simulink model "sistem_ver"  (R2020b)
settings: Solver=ode45  StartTime=0.0  StopTime=10  MaxStep=0.01  RelTol=1e-3
undefined symbols (not defined in the file or in its folder): K_d, K_p, params, r_des
settings Model: Creator=Danil  LastModifiedBy=Danil

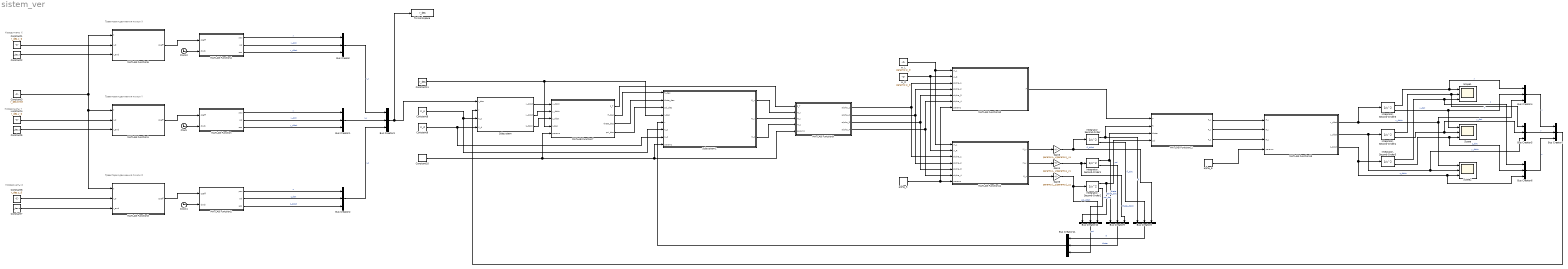
== system sistem_ver ==
  note: Траектория движения по оси Z
  note: Траектория движения по оси Y
  note: Координаты Y
  note: Траектория движения по оси X
  note: Координаты Z
  note: Координаты X
  Bus Creator{,1..11} (12 alike) : BusCreator  Inputs=3
  Clock : Clock
  Clock1 : Clock
  Clock2 : Clock
  Constant1 : Constant  Value=r_des.x_0
  Constant10 : Constant  Value=params  OutDataTypeStr=Bus: params_bus
  Constant11 : Constant  Value=r_des  OutDataTypeStr=Bus: r_des_bus
  Constant2 : Constant  Value=r_des.x
  Constant3 : Constant  Value=r_des.time
  Constant4 : Constant  Value=r_des.y_0
  Constant5 : Constant  Value=r_des.y
  Constant6 : Constant  Value=r_des.z_0
  Constant7 : Constant  Value=r_des.z
  Constant8 : Constant  Value=K_p  OutDataTypeStr=Bus: K_p_bus
  Constant9 : Constant  Value=K_d  OutDataTypeStr=Bus: K_d_bus
  Gain3 : Gain  Gain=params.L_x/params.J_xx
  Gain4 : Gain  Gain=params.L_y/params.J_yy
  Gain5 : Gain  Gain=params.L_z/params.J_zz
  Integrator, Second-Order{,1..5} (6 alike) : SecondOrderIntegrator
  MATLAB Function : MATLAB Function  TreatAsAtomicUnit=on
  MATLAB Function1 : MATLAB Function  TreatAsAtomicUnit=on
  MATLAB Function10 : MATLAB Function  TreatAsAtomicUnit=on
  MATLAB Function11 : MATLAB Function  TreatAsAtomicUnit=on
  MATLAB Function12 : MATLAB Function  TreatAsAtomicUnit=on
  MATLAB Function13 : MATLAB Function  TreatAsAtomicUnit=on
  MATLAB Function2 : MATLAB Function  TreatAsAtomicUnit=on
  MATLAB Function3 : MATLAB Function  TreatAsAtomicUnit=on
  MATLAB Function4 : MATLAB Function  TreatAsAtomicUnit=on
  MATLAB Function5 : MATLAB Function  TreatAsAtomicUnit=on
  MATLAB Function7 : MATLAB Function  TreatAsAtomicUnit=on
  MATLAB Function9 : MATLAB Function  TreatAsAtomicUnit=on
  Scope : Scope  NumInputPorts=3
  Scope1 : Scope  NumInputPorts=3
  Scope2 : Scope  NumInputPorts=3
  Subsystem : Subsystem
  Subsystem1 : Subsystem
  To Workspace : ToWorkspace  VariableName=r_des  SaveFormat=Timeseries  SampleTime=-1
  alpha_5 : Constant  Value=params  OutDataTypeStr=Bus: params_bus
  alpha_6 : Constant  Value=params  OutDataTypeStr=Bus: params_bus
  w_L : Constant  Value=params.w_0
  w_R : Constant  Value=params.w_0
  wires:
  MATLAB Function/3(acc) -> Bus Creator1/3  "y_ddot"
  Bus Creator/1 -> Bus Creator3/1  "r_x"
  MATLAB Function2/3(acc) -> Bus Creator2/3  "z_ddot"
  Bus Creator1/1 -> Bus Creator3/2  "r_y"
  Bus Creator2/1 -> Bus Creator3/3  "r_z"
  MATLAB Function3/1(coeff) -> MATLAB Function2/1(coeff)
  Clock/1 -> MATLAB Function/2(clock)
  Constant4/1 -> MATLAB Function1/2(r_0)
  Clock1/1 -> MATLAB Function2/2(clock)
  MATLAB Function1/1(coeff) -> MATLAB Function/1(coeff)
  Constant3/1 -> MATLAB Function3/1(t), MATLAB Function1/1(t), MATLAB Function5/1(t)
  Constant5/1 -> MATLAB Function1/3(r_end)
  Constant2/1 -> MATLAB Function5/3(r_end)
  Constant1/1 -> MATLAB Function5/2(r_0)
  MATLAB Function2/1(pos) -> Bus Creator2/1  "z"
  MATLAB Function/1(pos) -> Bus Creator1/1  "y"
  Constant7/1 -> MATLAB Function3/3(r_end)
  Constant6/1 -> MATLAB Function3/2(r_0)
  MATLAB Function/2(vel) -> Bus Creator1/2  "y_dot"
  MATLAB Function5/1(coeff) -> MATLAB Function4/1(coeff)
  Clock2/1 -> MATLAB Function4/2(clock)
  MATLAB Function4/2(vel) -> Bus Creator/2  "x_dot"
  MATLAB Function4/3(acc) -> Bus Creator/3  "x_ddot"
  MATLAB Function4/1(pos) -> Bus Creator/1  "x"
  MATLAB Function2/2(vel) -> Bus Creator2/2  "z_dot"
  MATLAB Function7/1(F_T) -> MATLAB Function9/1(F_T)
  Constant10/1 -> MATLAB Function7/5(params), Subsystem1/8(params), MATLAB Function9/5(params)
  "Integrator, Second-Order"/1 -> Bus Creator8/1, MATLAB Function12/2(fi)  "fi"
  MATLAB Function11/3(M_z) -> Gain5/1
  "Integrator, Second-Order2"/1 -> Bus Creator10/1, MATLAB Function12/4(psi)  "psi"
  "Integrator, Second-Order5"/2 -> Bus Creator6/2, Scope/3  "z_dot"
  Gain5/1 -> "Integrator, Second-Order2"/1, Bus Creator10/3  "psi_ddot"
  "Integrator, Second-Order4"/2 -> Bus Creator5/2, Scope/2  "y_dot"
  MATLAB Function11/2(M_y) -> Gain4/1
  w_R/1 -> MATLAB Function11/2(w_R), MATLAB Function10/2(w_R)
  "Integrator, Second-Order5"/1 -> Bus Creator6/1, Scope1/3  "z"
  MATLAB Function12/2(F_y) -> MATLAB Function13/2(F_y)
  MATLAB Function12/1(F_x) -> MATLAB Function13/1(F_x)
  "Integrator, Second-Order3"/2 -> Bus Creator4/2, Scope/1  "x_dot"
  MATLAB Function13/1(x_ddot) -> "Integrator, Second-Order3"/1, Bus Creator4/3, Scope2/1  "x_ddot"
  "Integrator, Second-Order3"/1 -> Bus Creator4/1, Scope1/1  "x"
  MATLAB Function13/3(z_ddot) -> Bus Creator6/3, Scope2/3, "Integrator, Second-Order5"/1  "z_ddot"
  MATLAB Function13/2(y_ddot) -> Bus Creator5/3, Scope2/2, "Integrator, Second-Order4"/1  "y_ddot"
  "Integrator, Second-Order1"/1 -> Bus Creator9/1, MATLAB Function12/3(theta)  "theta"
  MATLAB Function11/1(M_x) -> Gain3/1
  alpha_5/1 -> MATLAB Function10/7(params), MATLAB Function11/7(params)
  "Integrator, Second-Order4"/1 -> Bus Creator5/1, Scope1/2  "y"
  MATLAB Function9/3(alpha_3) -> MATLAB Function11/5(alpha_3), MATLAB Function10/5(alpha_3)
  alpha_6/1 -> MATLAB Function13/4(params)
  w_L/1 -> MATLAB Function10/1(w_L), MATLAB Function11/1(w_L)
  Gain3/1 -> Bus Creator8/3, "Integrator, Second-Order"/1  "fi_ddot"
  Gain4/1 -> Bus Creator9/3, "Integrator, Second-Order1"/1  "theta_ddot"
  MATLAB Function9/2(alpha_2) -> MATLAB Function11/4(alpha_2), MATLAB Function10/4(alpha_2)
  MATLAB Function9/1(alpha_1) -> MATLAB Function10/3(alpha_1), MATLAB Function11/3(alpha_1)
  MATLAB Function10/1(F) -> MATLAB Function12/1(F)
  MATLAB Function12/3(F_z) -> MATLAB Function13/3(F_z)
  MATLAB Function9/4(alpha_4) -> MATLAB Function11/6(alpha_4), MATLAB Function10/6(alpha_4)
  Constant8/1 -> Subsystem1/6(K_p), Subsystem/3(K_p)
  Constant9/1 -> Subsystem1/7(K_d), Subsystem/4(K_d)
  Bus Creator3/1 -> To Workspace/1, Subsystem/1(r_des)
  Constant11/1 -> MATLAB Function7/4(r_des), Subsystem1/4(r_des)
  "Integrator, Second-Order"/2 -> Bus Creator8/2  "fi_dot"
  "Integrator, Second-Order1"/2 -> Bus Creator9/2  "tehta_dot"
  "Integrator, Second-Order2"/2 -> Bus Creator10/2  "psi_dot"
  Bus Creator9/1 -> Bus Creator11/2  "theta"
  Bus Creator8/1 -> Bus Creator11/1  "fi"
  Bus Creator10/1 -> Bus Creator11/3  "psi"
  Bus Creator4/1 -> Bus Creator7/1  "x"
  Bus Creator5/1 -> Bus Creator7/2  "y"
  Bus Creator6/1 -> Bus Creator7/3  "z"
  Bus Creator7/1 -> Subsystem/2(r)
  Subsystem/1(x_ddot) -> MATLAB Function7/1(x_ddot)
  Subsystem/2(y_ddot) -> MATLAB Function7/2(y_ddot)
  Subsystem/3(z_ddot) -> MATLAB Function7/3(z_ddot)
  MATLAB Function7/2(fi_des) -> Subsystem1/1(fi_des)
  MATLAB Function7/3(theta_des) -> Subsystem1/2(theta_des)
  MATLAB Function7/4(psi_des) -> Subsystem1/3(psi_des)
  Bus Creator11/1 -> Subsystem1/5(r)
  Subsystem1/1(M_x) -> MATLAB Function9/2(M_x)
  Subsystem1/2(M_y) -> MATLAB Function9/3(M_y)
  Subsystem1/3(M_z) -> MATLAB Function9/4(M_z)

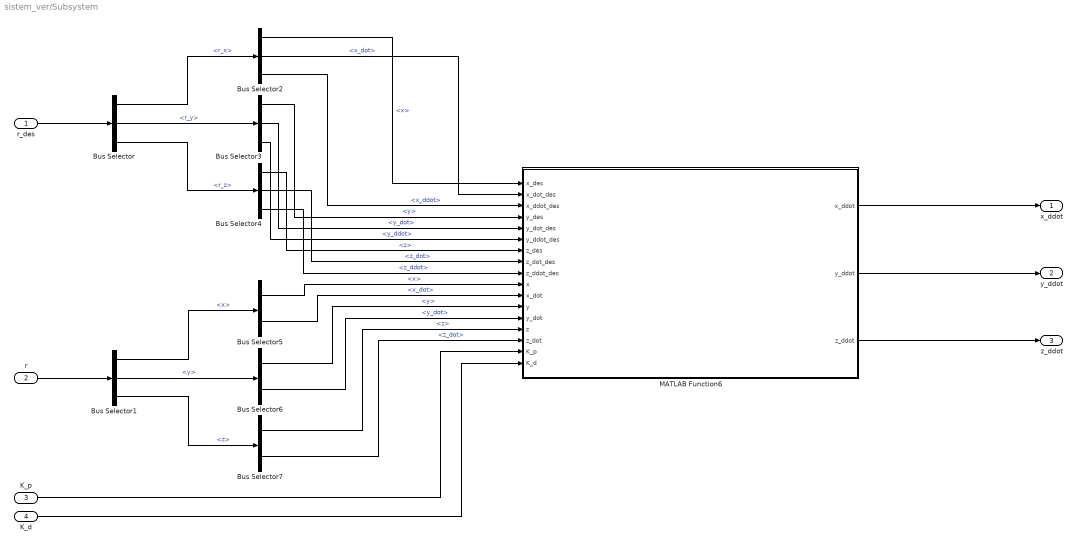
== system sistem_ver/Subsystem ==
  r_des : Inport
  r : Inport  Port=2
  K_p : Inport  Port=3
  K_d : Inport  Port=4
  Bus Selector : BusSelector  OutputSignals=r_x,r_y,r_z
  Bus Selector1 : BusSelector  OutputSignals=x,y,z
  Bus Selector2 : BusSelector  OutputSignals=x,x_dot,x_ddot
  Bus Selector3 : BusSelector  OutputSignals=y,y_dot,y_ddot
  Bus Selector4 : BusSelector  OutputSignals=z,z_dot,z_ddot
  Bus Selector5 : BusSelector  OutputSignals=x,x_dot
  Bus Selector6 : BusSelector  OutputSignals=y,y_dot
  Bus Selector7 : BusSelector  OutputSignals=z,z_dot
  MATLAB Function6 : MATLAB Function  TreatAsAtomicUnit=on
  x_ddot : Outport
  y_ddot : Outport  Port=2
  z_ddot : Outport  Port=3
  wires:
  MATLAB Function6/1(x_ddot) -> x_ddot/1
  MATLAB Function6/3(z_ddot) -> z_ddot/1
  K_p/1 -> MATLAB Function6/16(K_p)
  MATLAB Function6/2(y_ddot) -> y_ddot/1
  K_d/1 -> MATLAB Function6/17(K_d)
  r_des/1 -> Bus Selector/1
  r/1 -> Bus Selector1/1
  Bus Selector/1 -> Bus Selector2/1  "<r_x>"
  Bus Selector/2 -> Bus Selector3/1  "<r_y>"
  Bus Selector/3 -> Bus Selector4/1  "<r_z>"
  Bus Selector1/1 -> Bus Selector5/1  "<x>"
  Bus Selector1/2 -> Bus Selector6/1  "<y>"
  Bus Selector1/3 -> Bus Selector7/1  "<z>"
  Bus Selector2/1 -> MATLAB Function6/1(x_des)  "<x>"
  Bus Selector2/2 -> MATLAB Function6/2(x_dot_des)  "<x_dot>"
  Bus Selector2/3 -> MATLAB Function6/3(x_ddot_des)  "<x_ddot>"
  Bus Selector3/1 -> MATLAB Function6/4(y_des)  "<y>"
  Bus Selector3/2 -> MATLAB Function6/5(y_dot_des)  "<y_dot>"
  Bus Selector3/3 -> MATLAB Function6/6(y_ddot_des)  "<y_ddot>"
  Bus Selector4/1 -> MATLAB Function6/7(z_des)  "<z>"
  Bus Selector4/2 -> MATLAB Function6/8(z_dot_des)  "<z_dot>"
  Bus Selector4/3 -> MATLAB Function6/9(z_ddot_des)  "<z_ddot>"
  Bus Selector5/1 -> MATLAB Function6/10(x)  "<x>"
  Bus Selector5/2 -> MATLAB Function6/11(x_dot)  "<x_dot>"
  Bus Selector6/1 -> MATLAB Function6/12(y)  "<y>"
  Bus Selector6/2 -> MATLAB Function6/13(y_dot)  "<y_dot>"
  Bus Selector7/1 -> MATLAB Function6/14(z)  "<z>"
  Bus Selector7/2 -> MATLAB Function6/15(z_dot)  "<z_dot>"

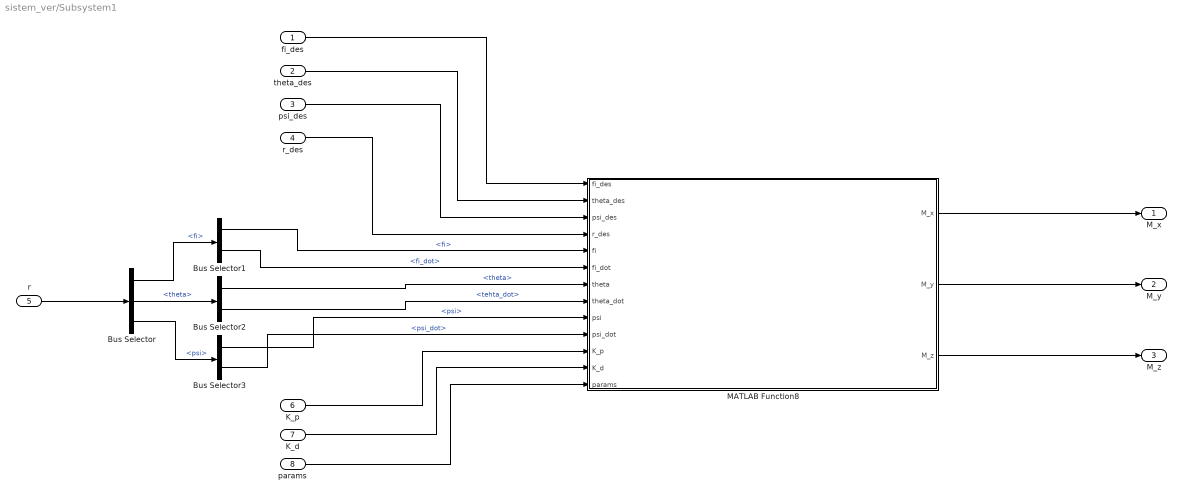
== system sistem_ver/Subsystem1 ==
  fi_des : Inport
  theta_des : Inport  Port=2
  psi_des : Inport  Port=3
  r_des : Inport  Port=4
  r : Inport  Port=5
  K_p : Inport  Port=6
  K_d : Inport  Port=7
  params : Inport  Port=8
  Bus Selector : BusSelector  OutputSignals=fi,theta,psi
  Bus Selector1 : BusSelector  OutputSignals=fi,fi_dot
  Bus Selector2 : BusSelector  OutputSignals=theta,tehta_dot
  Bus Selector3 : BusSelector  OutputSignals=psi,psi_dot
  MATLAB Function8 : MATLAB Function  TreatAsAtomicUnit=on
  M_x : Outport
  M_y : Outport  Port=2
  M_z : Outport  Port=3
  wires:
  MATLAB Function8/1(M_x) -> M_x/1
  params/1 -> MATLAB Function8/13(params)
  r_des/1 -> MATLAB Function8/4(r_des)
  psi_des/1 -> MATLAB Function8/3(psi_des)
  fi_des/1 -> MATLAB Function8/1(fi_des)
  theta_des/1 -> MATLAB Function8/2(theta_des)
  MATLAB Function8/2(M_y) -> M_y/1
  MATLAB Function8/3(M_z) -> M_z/1
  K_d/1 -> MATLAB Function8/12(K_d)
  K_p/1 -> MATLAB Function8/11(K_p)
  r/1 -> Bus Selector/1
  Bus Selector/1 -> Bus Selector1/1  "<fi>"
  Bus Selector/2 -> Bus Selector2/1  "<theta>"
  Bus Selector/3 -> Bus Selector3/1  "<psi>"
  Bus Selector1/1 -> MATLAB Function8/5(fi)  "<fi>"
  Bus Selector1/2 -> MATLAB Function8/6(fi_dot)  "<fi_dot>"
  Bus Selector2/1 -> MATLAB Function8/7(theta)  "<theta>"
  Bus Selector2/2 -> MATLAB Function8/8(theta_dot)  "<tehta_dot>"
  Bus Selector3/1 -> MATLAB Function8/9(psi)  "<psi>"
  Bus Selector3/2 -> MATLAB Function8/10(psi_dot)  "<psi_dot>"

== matlab function sistem_ver/MATLAB Function7 ==
  data: F_T output; fi_des output; x_ddot input; y_ddot input; z_ddot input; r_des input; params input; theta_des output; psi_des output
function [F_T, fi_des, theta_des, psi_des] = fcn(x_ddot, y_ddot, z_ddot, r_des, params)

F_T = params.m * (z_ddot + params.g);

fi_des = (1 / params.g) * (x_ddot * sin(r_des.psi) - y_ddot * cos(r_des.psi));
theta_des = (1 / params.g) * (x_ddot * cos(r_des.psi) + y_ddot * sin(r_des.psi));
psi_des = r_des.psi;

== matlab function sistem_ver/Subsystem1/MATLAB Function8 ==
  data: fi_des input; theta_des input; psi_des input; r_des input; fi input; fi_dot input; theta input; theta_dot input; psi input; psi_dot input; M_x output; K_p input; K_d input; params input; M_y output; M_z output
function [M_x, M_y, M_z] = fcn(fi_des, theta_des, psi_des, r_des, fi, fi_dot, theta, theta_dot, psi, psi_dot, K_p, K_d, params)

M_x = (params.J_xx / params.L_x) * (r_des.fi_ddot + abs(K_d.fi) * (r_des.fi_dot - fi_dot) + abs(K_p.fi) * (fi_des - fi));
M_y = (params.J_yy / params.L_y) * (r_des.theta_ddot + abs(K_d.theta) * (r_des.theta_dot - theta_dot) + abs(K_p.theta) * (theta_des - theta));
M_z = (params.J_zz / params.L_z) * (r_des.psi_ddot + abs(K_d.psi) * (r_des.psi_dot - psi_dot) + abs(K_p.psi) * (psi_des - psi));

== matlab function sistem_ver/MATLAB Function9 ==
  data: F_T input; alpha_1 output; M_x input; M_y input; M_z input; params input; alpha_2 output; alpha_3 output; alpha_4 output
function [alpha_1, alpha_2, alpha_3, alpha_4] = fcn(F_T, M_x, M_y, M_z, params)

alpha_1 = (1 / (4 * params.k_Y)) * (F_T + M_x + M_y + M_z) - 7;
alpha_2 = (1 / (4 * params.k_Y)) * (F_T + M_x - M_y - M_z);
alpha_3 = (1 / (4 * params.k_Y)) * (F_T - M_x + M_y - M_z) - 7;
alpha_4 = (1 / (4 * params.k_Y)) * (F_T - M_x - M_y + M_z);

== matlab function sistem_ver/MATLAB Function10 ==
  data: w_L input; F output; w_R input; alpha_1 input; alpha_2 input; alpha_3 input; alpha_4 input; params input
function F = fcn(w_L, w_R, alpha_1, alpha_2, alpha_3, alpha_4, params)
alpha_L = alpha_1 + alpha_2;
alpha_R = alpha_3 + alpha_4;

C_Y_L = 0.1545 * (alpha_L + 7);
C_Y_R = 0.1545 * (alpha_R + 7);

F = (3/2) * params.rho * params.S_l * (C_Y_L * w_L^2 + C_Y_R * w_R^2);

== matlab function sistem_ver/MATLAB Function11 ==
  data: w_L input; M_x output; w_R input; alpha_1 input; alpha_2 input; alpha_3 input; alpha_4 input; params input; M_y output; M_z output
function [M_x, M_y, M_z] = fcn(w_L, w_R, alpha_1, alpha_2, alpha_3, alpha_4, params)

%alpha_1 = alpha_1 * pi / 180;
%alpha_2 = alpha_2 * pi / 180;
%alpha_3 = alpha_3 * pi / 180;
%alpha_4 = alpha_4 * pi / 180;

%M_x = params.k_F * (w_L^2 * (alpha_1 + alpha_2) - w_R^2 * (alpha_3 + alpha_4));
%M_y = params.k_F * (w_L^2 * (alpha_1 - alpha_2) + w_R^2 * (alpha_3 - alpha_4));
%M_z = params.k_F * (w_L^2 * (alpha_1 - alpha_2) - w_R^2 * (alpha_3 - alpha_4));

M_x = (3/2) * params.rho * params.S_l * (0.1545 * ((alpha_1 + alpha_2) + 7) * w_L^2 - 0.1545 * ((alpha_3 + alpha_4) + 7) * w_R^2);
M_y = (3/2) * params.rho * params.S_l * (0.1545 * ((alpha_1 - alpha_2) + 7) * w_L^2 + 0.1545 * ((alpha_3 - alpha_4) + 7) * w_R^2);
M_z = (3/2) * params.rho * params.S_l * (0.1545 * ((alpha_1 - alpha_2) + 7) * w_L^2 - 0.1545 * ((alpha_3 - alpha_4) + 7) * w_R^2);

== matlab function sistem_ver/MATLAB Function12 ==
  data: F input; F_x output; fi input; theta input; psi input; F_y output; F_z output
function [F_x, F_y, F_z] = fcn(F, fi, theta, psi)

F_x = F * (cos(psi) * theta + fi * sin(psi));
F_y = F * (sin(psi) * theta - cos(psi) * fi);
F_z = F;

== matlab function sistem_ver/MATLAB Function13 ==
  data: F_x input; x_ddot output; F_y input; F_z input; params input; y_ddot output; z_ddot output
function [x_ddot, y_ddot, z_ddot] = fcn(F_x, F_y, F_z, params)

x_ddot = (1 / params.m) * F_x;
y_ddot = (1 / params.m) * F_y;
z_ddot = (1 / params.m) * (F_z - params.m * params.g);

== matlab function sistem_ver/MATLAB Function1 ==
  data: t input; coeff output; r_0 input; r_end input
function coeff  = calculation_coefficients(t, r_0, r_end)

x_0 = r_0;
x_dot_0 = 0;
x_ddot_0 = 0;

x_des = r_end;
x_dot_des = 0;
x_ddot_des = 0;

waypoints = [x_0    x_dot_0     x_ddot_0;
             x_des  x_dot_des   x_ddot_des]';
t = [0 t];

time_size = size(t);
n = 0;
%T = linspace(0, time_size(2) - 1, point(2));


border_conditions_sigm = reshape(waypoints(:, n + 1 : n + 2),1,[]);
%disp(border_conditions_sigm)

coeff = zeros(6, 1);

parameters = [1 * (t(n + 1) ^ 5), 1 * (t(n + 1) ^ 4), 1 * (t(n + 1) ^ 3), 1 * (t(n + 1) ^ 2), 1 * (t(n + 1) ^ 1), 1 * (t(n + 1) ^ 0);
              5 * (t(n + 1) ^ 4), 4 * (t(n + 1) ^ 3), 3 * (t(n + 1) ^ 2), 2 * (t(n + 1) ^ 1), 1 * (t(n + 1) ^ 0), 0 * (t(n + 1) ^ 0);
              20 * (t(n + 1) ^ 3), 12 * (t(n + 1) ^ 2), 6 * (t(n + 1) ^ 1), 2 * (t(n + 1) ^ 0), 0 * (t(n + 1) ^ 0), 0 * (t(n + 1) ^ 0);
              1 * (t(n + 2) ^ 5), 1 * (t(n + 2) ^ 4), 1 * (t(n + 2) ^ 3), 1 * (t(n + 2) ^ 2), 1 * (t(n + 2) ^ 1), 1 * (t(n + 2) ^ 0);
              5 * (t(n + 2) ^ 4), 4 * (t(n + 2) ^ 3), 3 * (t(n + 2) ^ 2), 2 * (t(n + 2) ^ 1), 1 * (t(n + 2) ^ 0), 0 * (t(n + 2) ^ 0);
              20 * (t(n + 2) ^ 3), 12 * (t(n + 2) ^ 2), 6 * (t(n + 2) ^ 1), 2 * (t(n + 2) ^ 0), 0 * (t(n + 2) ^ 0), 0 * (t(n + 2) ^ 0)];

coeff = inv(parameters) * border_conditions_sigm';

== matlab function sistem_ver/MATLAB Function ==
  data: coeff input; pos output; clock input; vel output; acc output
function [pos, vel, acc] = trajectories_calculation(coeff, clock)

T_p = [clock^5      clock^4     clock^3     clock^2     clock   1]';
T_v = [5*clock^4    4*clock^3   3*clock^2   2*clock     1       0]';
T_a = [20*clock^3   12*clock^2  6*clock     2           0       0]';

pos = sum(coeff.*T_p);
vel = sum(coeff.*T_v);
acc = sum(coeff.*T_a);

== matlab function sistem_ver/MATLAB Function2 ==
  data: coeff input; pos output; clock input; vel output; acc output
function [pos, vel, acc] = trajectories_calculation(coeff, clock)

T_p = [clock^5      clock^4     clock^3     clock^2     clock   1]';
T_v = [5*clock^4    4*clock^3   3*clock^2   2*clock     1       0]';
T_a = [20*clock^3   12*clock^2  6*clock     2           0       0]';

pos = sum(coeff.*T_p);
vel = sum(coeff.*T_v);
acc = sum(coeff.*T_a);

== matlab function sistem_ver/MATLAB Function3 ==
  data: t input; coeff output; r_0 input; r_end input
function coeff  = calculation_coefficients(t, r_0, r_end)

x_0 = r_0;
x_dot_0 = 0;
x_ddot_0 = 0;

x_des = r_end;
x_dot_des = 0;
x_ddot_des = 0;

waypoints = [x_0    x_dot_0     x_ddot_0;
             x_des  x_dot_des   x_ddot_des]';
t = [0 t];

time_size = size(t);
n = 0;
%T = linspace(0, time_size(2) - 1, point(2));


border_conditions_sigm = reshape(waypoints(:, n + 1 : n + 2),1,[]);
%disp(border_conditions_sigm)

coeff = zeros(6, 1);

parameters = [1 * (t(n + 1) ^ 5), 1 * (t(n + 1) ^ 4), 1 * (t(n + 1) ^ 3), 1 * (t(n + 1) ^ 2), 1 * (t(n + 1) ^ 1), 1 * (t(n + 1) ^ 0);
              5 * (t(n + 1) ^ 4), 4 * (t(n + 1) ^ 3), 3 * (t(n + 1) ^ 2), 2 * (t(n + 1) ^ 1), 1 * (t(n + 1) ^ 0), 0 * (t(n + 1) ^ 0);
              20 * (t(n + 1) ^ 3), 12 * (t(n + 1) ^ 2), 6 * (t(n + 1) ^ 1), 2 * (t(n + 1) ^ 0), 0 * (t(n + 1) ^ 0), 0 * (t(n + 1) ^ 0);
              1 * (t(n + 2) ^ 5), 1 * (t(n + 2) ^ 4), 1 * (t(n + 2) ^ 3), 1 * (t(n + 2) ^ 2), 1 * (t(n + 2) ^ 1), 1 * (t(n + 2) ^ 0);
              5 * (t(n + 2) ^ 4), 4 * (t(n + 2) ^ 3), 3 * (t(n + 2) ^ 2), 2 * (t(n + 2) ^ 1), 1 * (t(n + 2) ^ 0), 0 * (t(n + 2) ^ 0);
              20 * (t(n + 2) ^ 3), 12 * (t(n + 2) ^ 2), 6 * (t(n + 2) ^ 1), 2 * (t(n + 2) ^ 0), 0 * (t(n + 2) ^ 0), 0 * (t(n + 2) ^ 0)];

coeff = inv(parameters) * border_conditions_sigm';

== matlab function sistem_ver/MATLAB Function4 ==
  data: coeff input; pos output; clock input; vel output; acc output
function [pos, vel, acc] = trajectories_calculation(coeff, clock)

T_p = [clock^5      clock^4     clock^3     clock^2     clock   1]';
T_v = [5*clock^4    4*clock^3   3*clock^2   2*clock     1       0]';
T_a = [20*clock^3   12*clock^2  6*clock     2           0       0]';

pos = sum(coeff.*T_p);
vel = sum(coeff.*T_v);
acc = sum(coeff.*T_a);

== matlab function sistem_ver/MATLAB Function5 ==
  data: t input; coeff output; r_0 input; r_end input
function coeff  = calculation_coefficients(t, r_0, r_end)

x_0 = r_0;
x_dot_0 = 0;
x_ddot_0 = 0;

x_des = r_end;
x_dot_des = 0;
x_ddot_des = 0;

waypoints = [x_0    x_dot_0     x_ddot_0;
             x_des  x_dot_des   x_ddot_des]';
t = [0 t];

time_size = size(t);
n = 0;
%T = linspace(0, time_size(2) - 1, point(2));


border_conditions_sigm = reshape(waypoints(:, n + 1 : n + 2),1,[]);
%disp(border_conditions_sigm)

coeff = zeros(6, 1);

parameters = [1 * (t(n + 1) ^ 5), 1 * (t(n + 1) ^ 4), 1 * (t(n + 1) ^ 3), 1 * (t(n + 1) ^ 2), 1 * (t(n + 1) ^ 1), 1 * (t(n + 1) ^ 0);
              5 * (t(n + 1) ^ 4), 4 * (t(n + 1) ^ 3), 3 * (t(n + 1) ^ 2), 2 * (t(n + 1) ^ 1), 1 * (t(n + 1) ^ 0), 0 * (t(n + 1) ^ 0);
              20 * (t(n + 1) ^ 3), 12 * (t(n + 1) ^ 2), 6 * (t(n + 1) ^ 1), 2 * (t(n + 1) ^ 0), 0 * (t(n + 1) ^ 0), 0 * (t(n + 1) ^ 0);
              1 * (t(n + 2) ^ 5), 1 * (t(n + 2) ^ 4), 1 * (t(n + 2) ^ 3), 1 * (t(n + 2) ^ 2), 1 * (t(n + 2) ^ 1), 1 * (t(n + 2) ^ 0);
              5 * (t(n + 2) ^ 4), 4 * (t(n + 2) ^ 3), 3 * (t(n + 2) ^ 2), 2 * (t(n + 2) ^ 1), 1 * (t(n + 2) ^ 0), 0 * (t(n + 2) ^ 0);
              20 * (t(n + 2) ^ 3), 12 * (t(n + 2) ^ 2), 6 * (t(n + 2) ^ 1), 2 * (t(n + 2) ^ 0), 0 * (t(n + 2) ^ 0), 0 * (t(n + 2) ^ 0)];

coeff = inv(parameters) * border_conditions_sigm';

== matlab function sistem_ver/Subsystem/MATLAB Function6 ==
  data: x_des input; x_ddot output; x_dot_des input; x_ddot_des input; y_des input; y_dot_des input; y_ddot_des input; z_des input; z_dot_des input; z_ddot_des input; x input; x_dot input; y input; y_dot input; z input; z_dot input; K_p input; K_d input; y_ddot output; z_ddot output
function [x_ddot,y_ddot,z_ddot] = fcn(x_des, x_dot_des, x_ddot_des, y_des, y_dot_des, y_ddot_des, z_des, z_dot_des, z_ddot_des, ...
                                      x, x_dot, y, y_dot, z, z_dot, K_p, K_d)

x_ddot = x_ddot_des + abs(K_d.x) * (x_dot_des - x_dot) + abs(K_p.x) * (x_des - x);
y_ddot = y_ddot_des + abs(K_d.y) * (y_dot_des - y_dot) + abs(K_p.y) * (y_des - y);
z_ddot = z_ddot_des + abs(K_d.z) * (z_dot_des - z_dot) + abs(K_p.z) * (z_des - z);
